simulink model "Tank_based_Position_Position_discrete_kalman"  (R2020b)
settings: Solver=VariableStepAuto  StartTime=0.0  StopTime=50  RelTol=1e-3
values from neighbouring files (symbols this model uses):
  A = [1 Ts ... (first row only)    [parameters_Position_Position_kalman.m]
  alpha = 0.1    [parameters_Position_Position.m]    (also in parameters_Position_Position_kalman.m)
  Amp = 1    [parameters_Position_Position.m]    (also in parameters_Position_Position_kalman.m)
  Be = 10    [parameters_Position_Position.m]    (also in parameters_Position_Position_kalman.m)
  beta = 0.1    [parameters_Position_Position.m]    (also in parameters_Position_Position_kalman.m = 0.3)
  Bh = 1.5    [parameters_Position_Position.m]    (also in parameters_Position_Position_kalman.m)
  Bs = 200    [parameters_Position_Position.m]    (also in parameters_Position_Position_kalman.m)
  C = [1 0]    [parameters_Position_Position_kalman.m]
  delay = 1    [parameters_Position_Position.m]    (also in parameters_Position_Position_kalman.m)
  Dm = 0    [parameters_Position_Position.m]    (also in parameters_Position_Position_kalman.m)
  Ds = 0    [parameters_Position_Position.m]    (also in parameters_Position_Position_kalman.m)
  Fc = 0.5    [parameters_Position_Position.m]    (also in parameters_Position_Position_kalman.m)
  Fip = 100    [parameters_Position_Position.m]    (also in parameters_Position_Position_kalman.m)
  H_D = 1    [parameters_Position_Position.m]    (also in parameters_Position_Position_kalman.m)
  H_init_m = 1    [parameters_Position_Position.m]    (also in parameters_Position_Position_kalman.m = 20)
  H_init_s = 0    [parameters_Position_Position.m]    (also in parameters_Position_Position_kalman.m = 10)
  Ih = 2    [parameters_Position_Position.m]    (also in parameters_Position_Position_kalman.m)
  Je = 0    [parameters_Position_Position.m]    (also in parameters_Position_Position_kalman.m)
  Jh = 0    [parameters_Position_Position.m]    (also in parameters_Position_Position_kalman.m)
  Ke = 200    [parameters_Position_Position.m]    (also in parameters_Position_Position_kalman.m)
  Kh = 1    [parameters_Position_Position.m]    (also in parameters_Position_Position_kalman.m)
  Ks = 80    [parameters_Position_Position.m]    (also in parameters_Position_Position_kalman.m)
  Mm = 0.5    [parameters_Position_Position.m]    (also in parameters_Position_Position_kalman.m)
  Ms = 2    [parameters_Position_Position.m]    (also in parameters_Position_Position_kalman.m)
  Ph = 5    [parameters_Position_Position.m]    (also in parameters_Position_Position_kalman.m)
  R = 1    [parameters_Position_Position_kalman.m]
  tau = 100000    [parameters_Position_Position.m]    (also in parameters_Position_Position_kalman.m)
  Ts = 0.001    [parameters_Position_Position.m]    (also in parameters_Position_Position_kalman.m)
undefined symbols (not defined in the file or in its folder): DiscIntNeverNeededParam, Discrete, Time
libraries: simulink x4, ctrlSharedLib x2
settings Model: Creator=anuj  LastModifiedBy=Edoardo

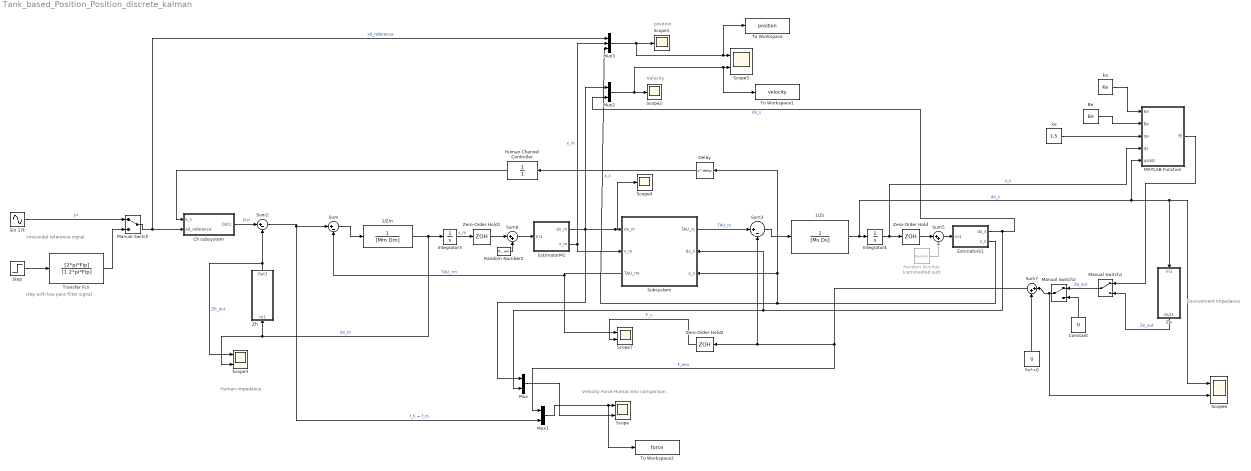
== system Tank_based_Position_Position_discrete_kalman ==
  note: Velocity
  note: position
  note: Environment Impedance
  note: Human impedance
  note: Velocity Force Human Env comparison
  note: sinusoidal reference signal
  note: step with low pass filter signal
  1/Zm : TransferFcn  Denominator=[Mm Dm]
  1/Zs : TransferFcn  Denominator=[Ms Ds]
  Be : Constant  Value=Be
  Ch subsystem : Subsystem
  Constant : Constant  Value=0
  Delay : Delay  DelayLength=delay  SampleTime=Ts
  EstimatorM1 : Subsystem
  EstimatorS1 : Subsystem
  Fe*=0 : Constant  Value=0
  Human Channel Controller : TransferFcn  Denominator=[1]
  Integrator3 : Integrator
  Integrator4 : Integrator
  MATLAB Function : MATLAB Function  TreatAsAtomicUnit=on
  Manual Switch : ManualSwitch
  Manual Switch1 : ManualSwitch
  Manual Switch2 : ManualSwitch
  Mux : Mux  Inputs=2
  Mux1 : Mux  Inputs=2
  Mux2 : Mux  Inputs=2
  Mux3 : Mux  Inputs=3
  Random Number : RandomNumber  Commented=on  Variance=0.000001  SampleTime=0.1
  Random Number2 : RandomNumber  Variance=0.000001  SampleTime=0.1
  Scope{,3,5..7} (5 alike) : Scope  NumInputPorts=2
  Scope1 : Scope
  Scope2 : Scope
  Scope4 : Scope
  Sin 17t : Sin  Amplitude=Amp  Frequency=Fc  SampleTime=0
  Step : Step  After=Amp  SampleTime=0
  Subsystem : Subsystem
      settings: PortSchema="{\"entries\":[{\"content\":{\"sides\":[{\"content\":{\"connectorIds\":[\"In1\",\"In2\",\"Out2\"]},\"type\":\"ConnectorPlacement.EquallySpacedRectSide\",\"uuid\":\"1b7528c3-158d-4350-af03-3a3e7550f0f6\"},{\"content\":{\"connectorIds\":[\"Out1\",\"In3\",\"In4\"],\"side\":\"RIGHT\"},\"type\":\"ConnectorPlacement.EquallySpacedRectSide\",\"uuid\":\"b309a382-b20d-41f2-81a6-a7afd0076f4c\"},{\"content\":{\"connectorIds\":[],\"side\":\"TOP\"},\"type\":\"ConnectorPlacement.EquallySpacedRectSide\",\"uuid\":\"571c96b8-da9a-48ed-ba7d-c86b8af7418f\"},{\"content\":{\"connectorIds\":[],\"side\":\"HIDDEN\"},\"type\":\"ConnectorPlacement.EquallySpacedRectSide\",\"uuid\":\"33f6671d-acb8-4428-b58d-b5b76ab6c677\"}]},\"type\":\"ConnectorPlacement.EquallySpacedConnector\",\"uuid\":\"aee86099-4484-4915-b829-1a330ba00ff1\"}],\"packageUris\":[\"http://schema.mathworks.com/mf0/Connector/R2020b\"],\"version\":\"1.0\"}"
  Sum : Sum  Inputs=|+-
  Sum2 : Sum  Inputs=|+-
  Sum3 : Sum  Inputs=|+-
  Sum5 : Sum  Inputs=|++
  Sum7 : Sum  Inputs=|++
  Sum8 : Sum  Inputs=|++
  To Workspace : ToWorkspace  VariableName=position  SaveFormat=Timeseries  SampleTime=-1
  To Workspace1 : ToWorkspace  VariableName=velocity  SaveFormat=Timeseries  SampleTime=-1
  To Workspace2 : ToWorkspace  VariableName=force  SaveFormat=Timeseries  SampleTime=-1
  Transfer Fcn : TransferFcn  Numerator=[2*pi*Fip]  Denominator=[1 2*pi*Fip]
  Ze : Subsystem
  Zero-Order Hold : ZeroOrderHold  SampleTime=Ts
  Zero-Order Hold1 : ZeroOrderHold  SampleTime=Ts
  Zero-Order Hold2 : ZeroOrderHold  SampleTime=-1
  Zh : Subsystem
  ke : Constant  Value=Ke
  xe : Constant  Value=1.5
  wires:
  Mux/1 -> Scope/2
  Mux1/1 -> To Workspace2/1, Scope/1
  Sum2/1 -> Sum/1, Mux1/2  "f_h = f_m"
  Subsystem/2(TAU_rm) -> Sum/2, Scope7/1  "TAU_rm"
  Fe*=0/1 -> Sum7/2
  Sum7/1 -> Mux1/1, Zero-Order Hold2/1, Sum3/2  "F_env"
  Ch subsystem/1(Out1) -> Sum2/1  "Fh*"
  Be/1 -> MATLAB Function/2(Be)
  xe/1 -> MATLAB Function/3(qe)
  ke/1 -> MATLAB Function/1(Ke)
  Transfer Fcn/1 -> Manual Switch/2
  Step/1 -> Transfer Fcn/1
  Human Channel Controller/1 -> Ch subsystem/1(x_s)
  Manual Switch/1 -> Mux3/1, Ch subsystem/2(xd_reference)  "xd_reference"
  Sin 17t/1 -> Manual Switch/1  "F*"
  MATLAB Function/1(fE) -> Manual Switch1/1
  Manual Switch1/1 -> Manual Switch2/1  "Ze_out"
  Zh/1(Out1) -> Sum2/2, Scope3/1  "Zh_out"
  Ze/1(Out1) -> Manual Switch1/2  "Ze_out"
  Mux2/1 -> Scope2/1, To Workspace1/1, Scope5/2
  Mux3/1 -> Scope1/1, To Workspace/1, Scope5/1
  Sum8/1 -> EstimatorM1/1(In1)
  Random Number2/1 -> Sum8/2
  1/Zm/1 -> Integrator3/1, Zh/1(In1), Scope3/2  "dx_m"
  Zero-Order Hold1/1 -> Sum8/1
  Integrator3/1 -> Zero-Order Hold1/1  "x_m"
  EstimatorM1/1(dx_m) -> Mux2/1, Mux/1, Scope4/1, Subsystem/1(dx_m)
  Sum5/1 -> EstimatorS1/1(In1)
  Random Number/1 -> Sum5/2
  Zero-Order Hold/1 -> Sum5/1
  Integrator4/1 -> Zero-Order Hold/1, MATLAB Function/4(qs)  "x_s"
  EstimatorS1/2(x_s) -> Delay/1, Subsystem/4(x_s), Mux3/3  "x_s"
  EstimatorS1/1(dx_s) -> Mux/2, Subsystem/3(dx_s), Mux2/2  "dx_s"
  1/Zs/1 -> Ze/1(In1), Scope6/1, MATLAB Function/5(qsdot), Integrator4/1  "dx_s"
  EstimatorM1/2(x_m) -> Subsystem/2(x_m), Mux3/2  "x_m"
  Zero-Order Hold2/1 -> Scope7/2  "F_s"
  Subsystem/1(TAU_rs) -> Sum3/1  "TAU_rs"
  Manual Switch2/1 -> Scope6/2, Sum7/1
  Constant/1 -> Manual Switch2/2
  Delay/1 -> Human Channel Controller/1
  Sum/1 -> 1/Zm/1
  Sum3/1 -> 1/Zs/1

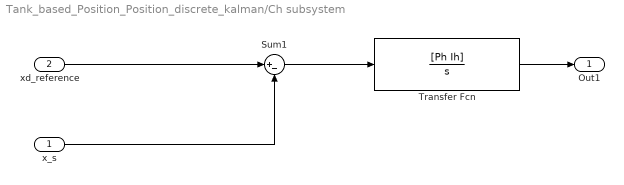
== system Tank_based_Position_Position_discrete_kalman/Ch subsystem ==
  x_s : Inport
  xd_reference : Inport  Port=2
  Sum1 : Sum  Inputs=|+-
  Transfer Fcn : TransferFcn  Numerator=[Ph Ih]  Denominator=[1 0]
  Out1 : Outport
  wires:
  x_s/1 -> Sum1/2
  Sum1/1 -> Transfer Fcn/1
  xd_reference/1 -> Sum1/1
  Transfer Fcn/1 -> Out1/1

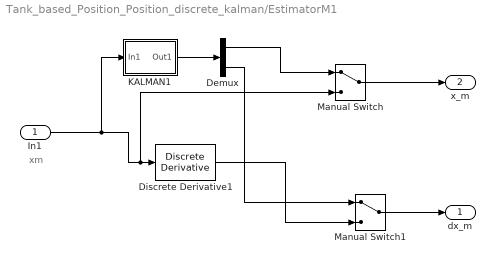
== system Tank_based_Position_Position_discrete_kalman/EstimatorM1 ==
  note: xm
  In1 : Inport
  Demux : Demux  Outputs=2
  Discrete Derivative1 : simulink/Discrete/Discrete Derivative  gainval=1.0  ICPrevScaledInput=0.0  OutMin=[]  OutMax=[]  OutDataType=fixdt(1, 16)  OutScaling=2^-10  DoSatur=off
  KALMAN1 : Subsystem
  Manual Switch : ManualSwitch
  Manual Switch1 : ManualSwitch
  dx_m : Outport
  x_m : Outport  Port=2
  wires:
  KALMAN1/1(Out1) -> Demux/1
  Demux/2 -> Manual Switch1/1
  Demux/1 -> Manual Switch/1
  Discrete Derivative1/1 -> Manual Switch1/2
  In1/1 -> KALMAN1/1(In1), Manual Switch/2, Discrete Derivative1/1
  Manual Switch1/1 -> dx_m/1
  Manual Switch/1 -> x_m/1

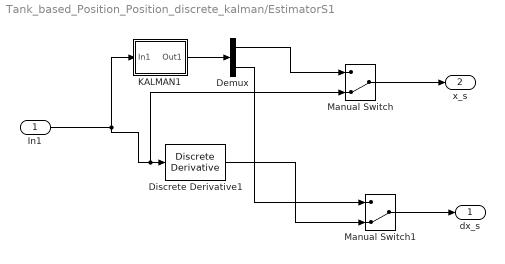
== system Tank_based_Position_Position_discrete_kalman/EstimatorS1 ==
  In1 : Inport
  Demux : Demux  Outputs=2
  Discrete Derivative1 : simulink/Discrete/Discrete Derivative  gainval=1.0  ICPrevScaledInput=0.0  OutMin=[]  OutMax=[]  OutDataType=fixdt(1, 16)  OutScaling=2^-10  DoSatur=off
  KALMAN1 : Subsystem
  Manual Switch : ManualSwitch  CurrentSetting=0
  Manual Switch1 : ManualSwitch  CurrentSetting=0
  dx_s : Outport
  x_s : Outport  Port=2
  wires:
  Manual Switch1/1 -> dx_s/1
  KALMAN1/1(Out1) -> Demux/1
  Demux/1 -> Manual Switch/1
  In1/1 -> Manual Switch/2, Discrete Derivative1/1, KALMAN1/1(In1)
  Discrete Derivative1/1 -> Manual Switch1/2
  Manual Switch/1 -> x_s/1
  Demux/2 -> Manual Switch1/1

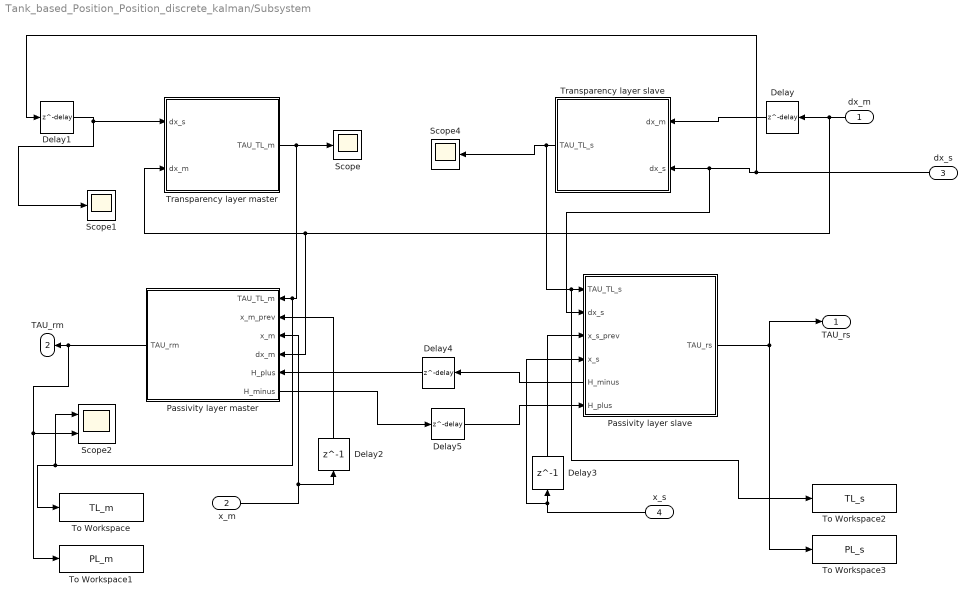
== system Tank_based_Position_Position_discrete_kalman/Subsystem ==
  dx_m : Inport
  x_m : Inport  Port=2
  dx_s : Inport  Port=3
  x_s : Inport  Port=4
  Delay{,1,4..5} (4 alike) : Delay  DelayLength=delay
  Delay2 : Delay  DelayLength=1
  Delay3 : Delay  DelayLength=1
  Passivity layer master : Subsystem
      settings: PortSchema="{\"entries\":[{\"content\":{\"sides\":[{\"content\":{\"connectorIds\":[\"Out2\"]},\"type\":\"ConnectorPlacement.EquallySpacedRectSide\",\"uuid\":\"110529f1-1521-4c75-adcc-f6b573829d74\"},{\"content\":{\"connectorIds\":[\"In1\",\"In2\",\"In3\",\"In4\",\"In5\",\"Out1\"],\"side\":\"RIGHT\"},\"type\":\"ConnectorPlacement.EquallySpacedRectSide\",\"uuid\":\"1063a40f-ea92-45b6-8f85-7c32271dcf13\"},{\"content\":{\"connectorIds\":[],\"side\":\"TOP\"},\"type\":\"ConnectorPlacement.EquallySpacedRectSide\",\"uuid\":\"a693b80b-d539-4e24-8520-20a85bf9095f\"},{\"content\":{\"connectorIds\":[],\"side\":\"HIDDEN\"},\"type\":\"ConnectorPlacement.EquallySpacedRectSide\",\"uuid\":\"257b4aaf-b283-4ddc-9c41-cf1bae620795\"}]},\"type\":\"ConnectorPlacement.EquallySpacedConnector\",\"uuid\":\"9fc20ba4-9e26-48d3-8eef-bb993afdd8a0\"}],\"packageUris\":[\"http://schema.mathworks.com/mf0/Connector/R2020b\"],\"version\":\"1.0\"}"
  Passivity layer slave : Subsystem
      settings: PortSchema="{\"entries\":[{\"content\":{\"sides\":[{\"content\":{\"connectorIds\":[\"In1\",\"In2\",\"In3\",\"In4\",\"Out2\",\"In5\"]},\"type\":\"ConnectorPlacement.EquallySpacedRectSide\",\"uuid\":\"110529f1-1521-4c75-adcc-f6b573829d74\"},{\"content\":{\"connectorIds\":[\"Out1\"],\"side\":\"RIGHT\"},\"type\":\"ConnectorPlacement.EquallySpacedRectSide\",\"uuid\":\"1063a40f-ea92-45b6-8f85-7c32271dcf13\"},{\"content\":{\"connectorIds\":[],\"side\":\"TOP\"},\"type\":\"ConnectorPlacement.EquallySpacedRectSide\",\"uuid\":\"a693b80b-d539-4e24-8520-20a85bf9095f\"},{\"content\":{\"connectorIds\":[],\"side\":\"HIDDEN\"},\"type\":\"ConnectorPlacement.EquallySpacedRectSide\",\"uuid\":\"257b4aaf-b283-4ddc-9c41-cf1bae620795\"}]},\"type\":\"ConnectorPlacement.EquallySpacedConnector\",\"uuid\":\"9fc20ba4-9e26-48d3-8eef-bb993afdd8a0\"}],\"packageUris\":[\"http://schema.mathworks.com/mf0/Connector/R2020b\"],\"version\":\"1.0\"}"
  Scope : Scope
  Scope1 : Scope
  Scope2 : Scope  NumInputPorts=2
  Scope4 : Scope
  To Workspace : ToWorkspace  VariableName=TL_m  SaveFormat=Timeseries  SampleTime=-1
  To Workspace1 : ToWorkspace  VariableName=PL_m  SaveFormat=Timeseries  SampleTime=-1
  To Workspace2 : ToWorkspace  VariableName=TL_s  SaveFormat=Timeseries  SampleTime=-1
  To Workspace3 : ToWorkspace  VariableName=PL_s  SaveFormat=Timeseries  SampleTime=-1
  Transparency layer master : Subsystem
  Transparency layer slave : Subsystem
  TAU_rs : Outport
  TAU_rm : Outport  Port=2
  wires:
  dx_m/1 -> Transparency layer master/2(dx_m), Passivity layer master/4(dx_m), Delay/1
  dx_s/1 -> Delay1/1, Passivity layer slave/2(dx_s), Transparency layer slave/2(dx_s)
  Delay1/1 -> Scope1/1, Transparency layer master/1(dx_s)
  Delay/1 -> Transparency layer slave/1(dx_m)
  Transparency layer master/1(TAU_TL_m) -> To Workspace/1, Scope2/1, Passivity layer master/1(TAU_TL_m), Scope/1
  Transparency layer slave/1(TAU_TL_s) -> To Workspace2/1, Passivity layer slave/1(TAU_TL_s), Scope4/1
  Passivity layer slave/2("\tH_minus") -> Delay4/1
  Passivity layer master/1(H_minus) -> Delay5/1
  x_m/1 -> Passivity layer master/3(x_m), Delay2/1
  Delay2/1 -> Passivity layer master/2(x_m_prev)
  x_s/1 -> Passivity layer slave/4(x_s), Delay3/1
  Delay3/1 -> Passivity layer slave/3(x_s_prev)
  Delay4/1 -> Passivity layer master/5(H_plus)
  Delay5/1 -> Passivity layer slave/5(H_plus)
  Passivity layer master/2(TAU_rm) -> To Workspace1/1, Scope2/2, TAU_rm/1
  Passivity layer slave/1(TAU_rs) -> To Workspace3/1, TAU_rs/1

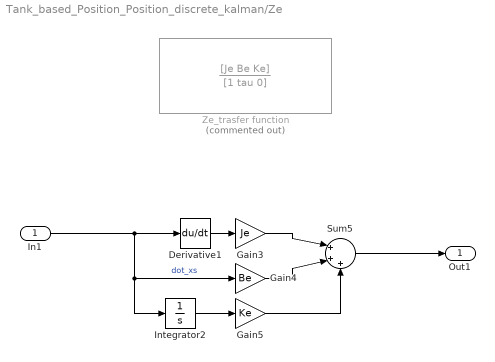
== system Tank_based_Position_Position_discrete_kalman/Ze ==
  In1 : Inport
  Derivative1 : Derivative
  Gain3 : Gain  Gain=Je
  Gain4 : Gain  Gain=Be
  Gain5 : Gain  Gain=Ke
  Integrator2 : Integrator
  Sum5 : Sum  Inputs=|+++
  Ze_trasfer function : TransferFcn  Commented=on  Numerator=[Je Be Ke]  Denominator=[1 tau 0]
  Out1 : Outport
  wires:
  Gain4/1 -> Sum5/2
  Gain3/1 -> Sum5/1
  Gain5/1 -> Sum5/3
  Sum5/1 -> Out1/1
  Integrator2/1 -> Gain5/1
  In1/1 -> Integrator2/1, Gain4/1, Derivative1/1  "dot_xs"
  Derivative1/1 -> Gain3/1

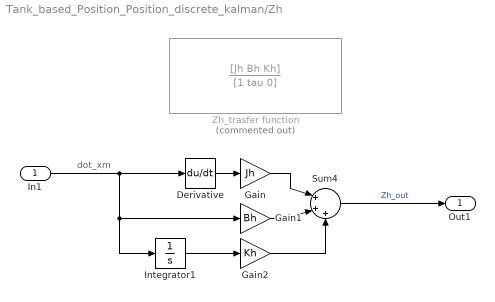
== system Tank_based_Position_Position_discrete_kalman/Zh ==
  note: dot_xm
  In1 : Inport
  Derivative : Derivative
  Gain : Gain  Gain=Jh
  Gain1 : Gain  Gain=Bh
  Gain2 : Gain  Gain=Kh
  Integrator1 : Integrator
  Sum4 : Sum  Inputs=|+++
  Zh_trasfer function : TransferFcn  Commented=on  Numerator=[Jh Bh Kh]  Denominator=[1 tau 0]
  Out1 : Outport
  wires:
  Derivative/1 -> Gain/1
  Integrator1/1 -> Gain2/1
  Gain2/1 -> Sum4/3
  Gain1/1 -> Sum4/2
  Gain/1 -> Sum4/1
  Sum4/1 -> Out1/1  "Zh_out"
  In1/1 -> Gain1/1, Integrator1/1, Derivative/1

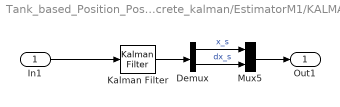
== system Tank_based_Position_Position_discrete_kalman/EstimatorM1/KALMAN1 ==
  In1 : Inport
  Demux : Demux  Outputs=2
  Kalman Filter : ctrlSharedLib/Kalman Filter  TimeDomain=Discrete-Time  UseCurrentEstimator=off  ModelSource=Individual A, B, C, D matrices  ModelSourceVariable=ss(0.95,1,1,0,1)  A=A  B=0  C=C  D=0  NumberOfStates=1  NumberOfInputs=1  NumberOfOutputs=1  InitialEstimateSource=Dialog  X0=0  P0=10  UseK=off  UseGH=off  NumberOfProcessNoiseInputs=1  G=1  TimeInvariantG=on  H=0  TimeInvariantH=on  Q=Q  TimeInvariantQ=on  R=R  TimeInvariantR=on  N=0  TimeInvariantN=on  AddInputPort=off  AddEnablePort=off  OutputEstimatedY=off  OutputP=off  Ts=Ts
  Mux5 : Mux  Inputs=2
  Out1 : Outport
  wires:
  Demux/1 -> Mux5/1  "x_s"
  Demux/2 -> Mux5/2  "dx_s"
  Kalman Filter/1 -> Demux/1
  Mux5/1 -> Out1/1
  In1/1 -> Kalman Filter/1

== system Tank_based_Position_Position_discrete_kalman/EstimatorS1/KALMAN1 ==
  In1 : Inport
  Demux : Demux  Outputs=2
  Kalman Filter : ctrlSharedLib/Kalman Filter  TimeDomain=Discrete-Time  UseCurrentEstimator=off  ModelSource=Individual A, B, C, D matrices  ModelSourceVariable=ss(0.95,1,1,0,1)  A=A  B=0  C=C  D=0  NumberOfStates=1  NumberOfInputs=1  NumberOfOutputs=1  InitialEstimateSource=Dialog  X0=0  P0=10  UseK=off  UseGH=off  NumberOfProcessNoiseInputs=1  G=1  TimeInvariantG=on  H=0  TimeInvariantH=on  Q=Q  TimeInvariantQ=on  R=R  TimeInvariantR=on  N=0  TimeInvariantN=on  AddInputPort=off  AddEnablePort=off  OutputEstimatedY=off  OutputP=off  Ts=Ts
  Mux5 : Mux  Inputs=2
  Out1 : Outport
  wires:
  Demux/1 -> Mux5/1  "x_s"
  Demux/2 -> Mux5/2  "dx_s"
  Kalman Filter/1 -> Demux/1
  Mux5/1 -> Out1/1
  In1/1 -> Kalman Filter/1

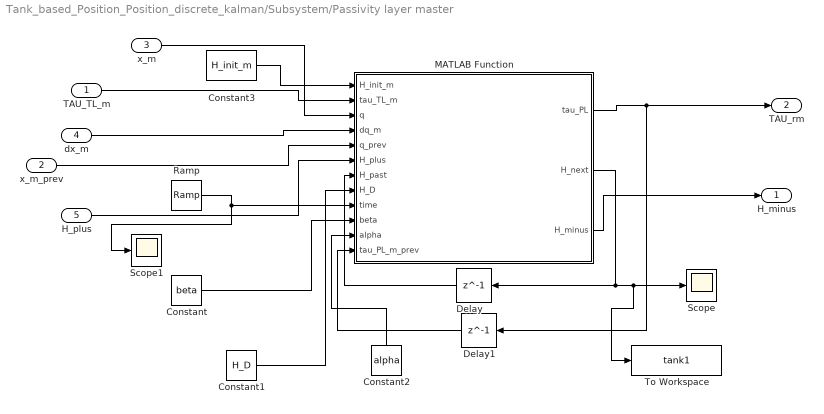
== system Tank_based_Position_Position_discrete_kalman/Subsystem/Passivity layer master ==
  TAU_TL_m : Inport
  x_m_prev : Inport  Port=2
  x_m : Inport  Port=3
  dx_m : Inport  Port=4
  H_plus : Inport  Port=5
  Constant : Constant  Value=beta
  Constant1 : Constant  Value=H_D
  Constant2 : Constant  Value=alpha
  Constant3 : Constant  Value=H_init_m
  Delay : Delay  DelayLength=1  InitialCondition=0
  Delay1 : Delay  DelayLength=1
  MATLAB Function : MATLAB Function  TreatAsAtomicUnit=on
  Ramp : simulink/Sources/Ramp  slope=1  start=0  InitialOutput=0
  Scope : Scope
  Scope1 : Scope
  To Workspace : ToWorkspace  VariableName=tank1  SaveFormat=Timeseries  SampleTime=-1
  H_minus : Outport
  TAU_rm : Outport  Port=2
  wires:
  MATLAB Function/1(tau_PL) -> Delay1/1, TAU_rm/1
  TAU_TL_m/1 -> MATLAB Function/2(tau_TL_m)
  H_plus/1 -> MATLAB Function/6(H_plus)
  MATLAB Function/2(H_next) -> Delay/1, To Workspace/1, Scope/1
  MATLAB Function/3(H_minus) -> H_minus/1
  dx_m/1 -> MATLAB Function/4(dq_m)
  x_m_prev/1 -> MATLAB Function/5(q_prev)
  x_m/1 -> MATLAB Function/3(q)
  Constant/1 -> MATLAB Function/10(beta)
  Constant1/1 -> MATLAB Function/8(H_D)
  Constant2/1 -> MATLAB Function/11(alpha)
  Delay/1 -> MATLAB Function/7(H_past)
  Ramp/1 -> Scope1/1, MATLAB Function/9(time)
  Delay1/1 -> MATLAB Function/12(tau_PL_m_prev)
  Constant3/1 -> MATLAB Function/1(H_init_m)

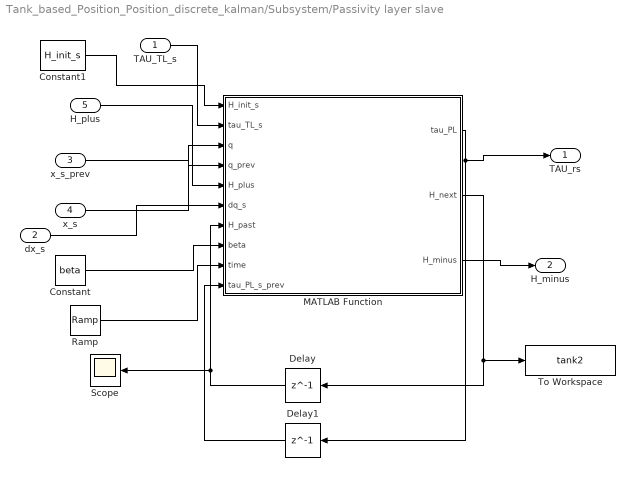
== system Tank_based_Position_Position_discrete_kalman/Subsystem/Passivity layer slave ==
  TAU_TL_s : Inport
  dx_s : Inport  Port=2
  x_s_prev : Inport  Port=3
  x_s : Inport  Port=4
  H_plus : Inport  Port=5
  Constant : Constant  Value=beta
  Constant1 : Constant  Value=H_init_s
  Delay : Delay  DelayLength=1  InitialCondition=0
  Delay1 : Delay  DelayLength=1
  MATLAB Function : MATLAB Function  TreatAsAtomicUnit=on
  Ramp : simulink/Sources/Ramp  slope=1  start=0  InitialOutput=0
  Scope : Scope
  To Workspace : ToWorkspace  VariableName=tank2  SaveFormat=Timeseries  SampleTime=-1
  TAU_rs : Outport
  "\tH_minus" : Outport  Port=2
  wires:
  MATLAB Function/1(tau_PL) -> Delay1/1, TAU_rs/1
  MATLAB Function/3(H_minus) -> "\tH_minus"/1
  MATLAB Function/2(H_next) -> To Workspace/1, Delay/1
  Delay/1 -> MATLAB Function/7(H_past), Scope/1
  H_plus/1 -> MATLAB Function/5(H_plus)
  x_s_prev/1 -> MATLAB Function/4(q_prev)
  x_s/1 -> MATLAB Function/3(q)
  Constant/1 -> MATLAB Function/8(beta)
  TAU_TL_s/1 -> MATLAB Function/2(tau_TL_s)
  Delay1/1 -> MATLAB Function/10(tau_PL_s_prev)
  Ramp/1 -> MATLAB Function/9(time)
  dx_s/1 -> MATLAB Function/6(dq_s)
  Constant1/1 -> MATLAB Function/1(H_init_s)

== system Tank_based_Position_Position_discrete_kalman/Subsystem/Transparency layer master ==
  dx_s : Inport
  dx_m : Inport  Port=2
  Cs : Subsystem
  Sum6 : Sum  Inputs=|-+
  TAU_TL_m : Outport
  wires:
  dx_m/1 -> Sum6/2  "dx_m"
  Cs/1(dx_s) -> TAU_TL_m/1
  Sum6/1 -> Cs/1(err)
  dx_s/1 -> Sum6/1  "dx_s"

== system Tank_based_Position_Position_discrete_kalman/Subsystem/Transparency layer slave ==
  dx_m : Inport
  dx_s : Inport  Port=2
  Cs : Subsystem
  Sum6 : Sum  Inputs=|+-
  TAU_TL_s : Outport
  wires:
  Sum6/1 -> Cs/1(err)
  dx_s/1 -> Sum6/2  "dx_s"
  dx_m/1 -> Sum6/1  "dx_m"
  Cs/1(dx_s) -> TAU_TL_s/1

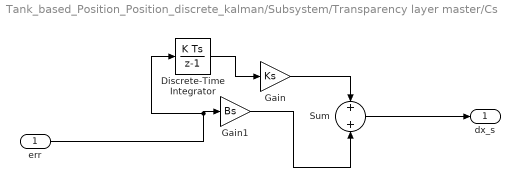
== system Tank_based_Position_Position_discrete_kalman/Subsystem/Transparency layer master/Cs ==
  err : Inport
  Discrete-Time Integrator : DiscreteIntegrator  SampleTime=Ts  ICPrevOutput=DiscIntNeverNeededParam  ICPrevScaledInput=DiscIntNeverNeededParam
  Gain : Gain  Gain=Ks
  Gain1 : Gain  Gain=Bs
  Sum : Sum
  dx_s : Outport
  wires:
  Gain1/1 -> Sum/2
  err/1 -> Discrete-Time Integrator/1, Gain1/1
  Discrete-Time Integrator/1 -> Gain/1
  Gain/1 -> Sum/1
  Sum/1 -> dx_s/1

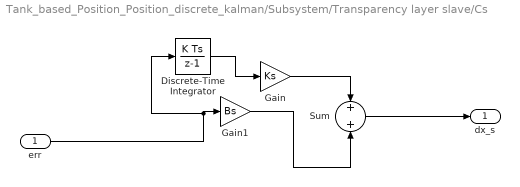
== system Tank_based_Position_Position_discrete_kalman/Subsystem/Transparency layer slave/Cs ==
  err : Inport
  Discrete-Time Integrator : DiscreteIntegrator  SampleTime=Ts  ICPrevOutput=DiscIntNeverNeededParam  ICPrevScaledInput=DiscIntNeverNeededParam
  Gain : Gain  Gain=Ks
  Gain1 : Gain  Gain=Bs
  Sum : Sum
  dx_s : Outport
  wires:
  Gain1/1 -> Sum/2
  err/1 -> Discrete-Time Integrator/1, Gain1/1
  Discrete-Time Integrator/1 -> Gain/1
  Gain/1 -> Sum/1
  Sum/1 -> dx_s/1

== matlab function Tank_based_Position_Position_discrete_kalman/Subsystem/Passivity layer master/MATLAB Function ==
  data: H_init_m input; tau_TL_m input; tau_PL output; H_next output; H_minus output; q input; dq_m input; q_prev input; H_plus input; H_past input; H_D input; time input; beta input; alpha input; tau_PL_m_prev input
function [tau_PL, H_next, H_minus] = Passivity_layer(H_init_m, tau_TL_m, q, dq_m, q_prev, H_plus, H_past, H_D, time, beta, alpha, tau_PL_m_prev)

% init
Ts = 0.001;
if time == 0
    H_past = H_init_m;
    tau_PL_m_prev = 0; 
end

delta_HI = tau_PL_m_prev*(q - q_prev);
H = H_past + H_plus - delta_HI;

% compute tau max 1
if H <= 0 
    tau_max_1 = 0;
else
    tau_max_1 = tau_TL_m;
end

% compute tau max 2
if abs(dq_m) < 0.01
    tau_max_2 = sign(dq_m)*10000;
else
    tau_max_2 =  H/(dq_m*Ts);
end

% compute tau_PL
tau_PL = sign(tau_TL_m)*min(abs(tau_max_1),abs(tau_max_2));

if(H < H_D)
   d = alpha*(H_D - H);
   tau_TLC = -d*dq_m;
   tau_PL = tau_PL + tau_TLC;
end

H_minus = beta*H;
H_next = H - H_minus;

== matlab function Tank_based_Position_Position_discrete_kalman/MATLAB Function ==
  data: Ke input; fE output; Be input; qe input; qs input; qsdot input
function fE = environment(Ke, Be, qe, qs, qsdot)
    if qs > qe
        fE = Ke * (qs - qe) + Be * qsdot;
    else
        fE = 0;
    end
end

== matlab function Tank_based_Position_Position_discrete_kalman/Subsystem/Passivity layer slave/MATLAB Function ==
  data: H_init_s input; tau_TL_s input; tau_PL output; q input; q_prev input; H_plus input; dq_s input; H_past input; H_next output; H_minus output; beta input; time input; tau_PL_s_prev input
function [tau_PL, H_next, H_minus] = Passivity_layer(H_init_s, tau_TL_s, q, q_prev, H_plus, dq_s, H_past, beta, time, tau_PL_s_prev)

% init
Ts = 0.001;
if time == 0
    H_past = H_init_s;
    tau_PL_s_prev = 0; 
end

delta_HI = tau_PL_s_prev*(q - q_prev);
H = H_past + H_plus - delta_HI;

% compute tau max 1
if H <= 0 
    tau_max_1 = 0;
else
    tau_max_1 = tau_TL_s;
end

% compute tau max 2
tau_max_2 =  H/(dq_s*Ts);


% compute tau_PL
tau_PL = sign(tau_TL_s)*min(abs(tau_max_1),abs(tau_max_2));


H_minus = beta*H;
H_next = H - H_minus;
